simulink model "Motor_Test_All"  (R2015b)
settings: Solver=FixedStepAuto  StartTime=0.0  StopTime=100.0  RelTol=1e-3
libraries: simulink x1
settings Model: SimulationMode=external  ExtModeTrigDuration=2  Creator=Joern  LastModifiedBy=Joern
settings OptimizationCC: OptimizeModelRefInitCode=on  LifeSpan=1  MaxStackSize=64
settings HardwareCC: ProdBitPerInt=16  ProdBitPerPointer=16  ProdLargestAtomicFloat=None  ProdWordSize=8  ProdHWDeviceType=Atmel->AVR
settings ModelReferenceCC: ParallelModelReferenceMATLABWorkerInit=Load Top Model
settings RTWCC: SystemTargetFile=ert.tlc  TemplateMakefile=ert_default_tmf  Description=Embedded Coder  Toolchain=Arduino AVR v1.6.1  BuildConfiguration=Faster Runs
settings CodeAppCC: IgnoreCustomStorageClasses=off
settings ERTTargetCC: GenerateSampleERTMain=on  SupportContinuousTime=on  SupportVariableSizeSignals=on

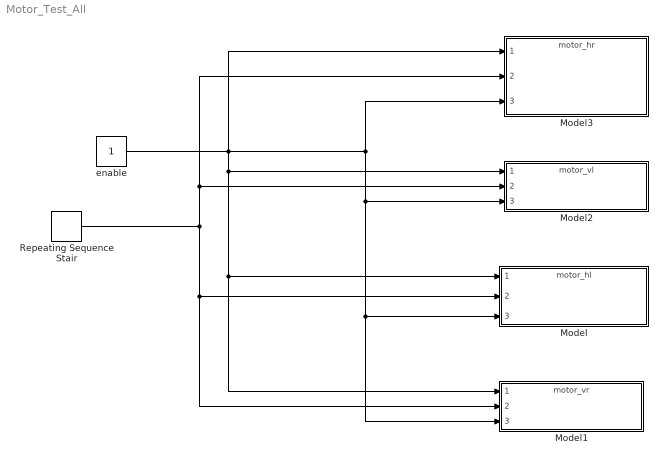
== system Motor_Test_All ==
  Model : ModelReference  ModelNameDialog=motor_hl.slx  SimulationMode=Normal  ModelReferenceVersion=1.4  CopyOfModelName=motor_hl.slx
  Model1 : ModelReference  ModelNameDialog=motor_vr.slx  SimulationMode=Normal  ModelReferenceVersion=1.4  CopyOfModelName=motor_vr.slx
  Model2 : ModelReference  ModelNameDialog=motor_vl.slx  SimulationMode=Normal  ModelReferenceVersion=1.4  CopyOfModelName=motor_vl.slx
  Model3 : ModelReference  ModelNameDialog=motor_hr.slx  SimulationMode=Normal  ModelReferenceVersion=1.6  CopyOfModelName=motor_hr.slx
  Repeating Sequence Stair : simulink/Sources/Repeating Sequence Stair  OutValues=[0 50 100 150 200 255 200 150 100 50 0 0 0 0 0 0 0 0].'  tsamp=10  OutMin=[]  OutMax=[]  OutDataTypeStr=double  OutputDataTypeScalingMode=double  OutDataType=fixdt(0,8)  ConRadixGroup=Best Precision: Vector-wise  OutScaling=2^-12
  enable : Constant
  wires:
  Repeating Sequence Stair/1 -> Model2/2, Model3/2, Model1/2, Model/2
  enable/1 -> Model1/3, Model/3, Model2/3, Model3/3, Model3/1, Model1/1, Model/1, Model2/1
